simulink model "pneumatic_tank_PI"  (R2021a)
settings: Solver=VariableStepAuto  StartTime=0.0  StopTime=16  RelTol=1e-3
model workspace (MATLAB code in the model file):
  | V = 0.4; %liter
  | alpha = 1.5/3;
  | p_s = 6; % bar
values from neighbouring files (symbols this model uses):
  a = (Phi'*Phi)^(-1)*Phi'*p_dot    [sysid_tank.m]
  K = 2.62    [tank_valve_PI_design.m]
  p0 = 2.5    [tank_valve_PI_design.m]
undefined symbols (not defined in the file or in its folder): b, tau_i
settings Model: Creator=kjartan  LastModifiedBy=kjartan
settings SolverCC: AlgebraicLoopSolver=TrustRegion
settings DataIOCC: ReturnWorkspaceOutputs=off
settings DebuggingCC: SFMachineParentedDataDiag=warning  ArithmeticOperatorsInVariantConditions=warning
settings SFSimCC: CustomCodeUndefinedFunction=UseInterfaceOnly

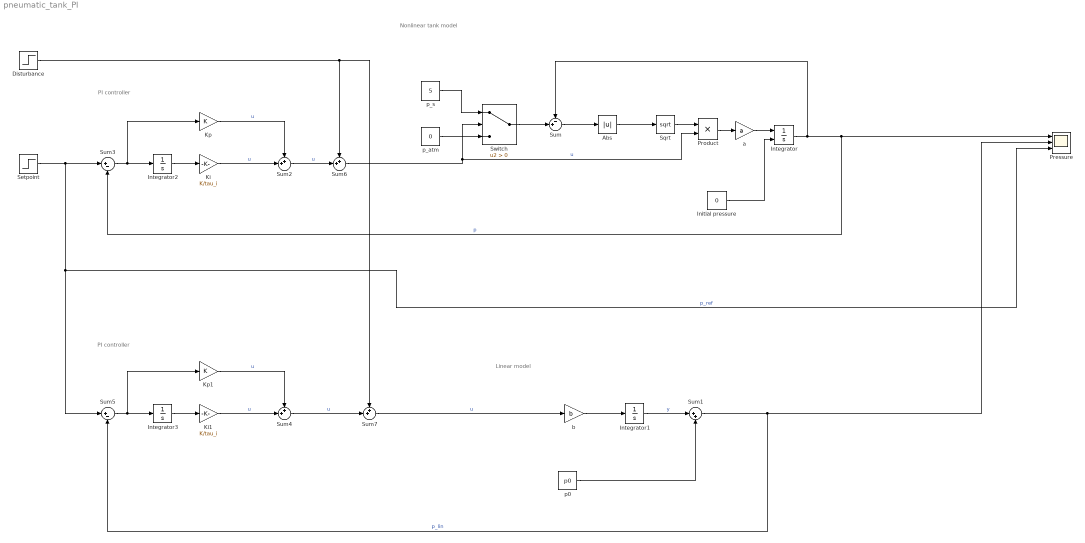
== system pneumatic_tank_PI ==
  note: PI controller
  note: PI controller
  note: Linear model
  note: Nonlinear tank model
  Abs : Abs
  Disturbance : Step  Time=10  SampleTime=0
  Initial pressure : Constant  Value=0  OutDataTypeStr=Inherit: Inherit via back propagation
  Integrator : Integrator  InitialConditionSource=external  InitialCondition=1  LimitOutput=on  LowerSaturationLimit=0
  Integrator1 : Integrator
  Integrator2 : Integrator
  Integrator3 : Integrator
  Ki : Gain  Gain=K/tau_i
  Ki1 : Gain  Gain=K/tau_i
  Kp : Gain  Gain=K
  Kp1 : Gain  Gain=K
  Pressure : Scope  NumInputPorts=3
  Product : Product
  Setpoint : Step  Time=2  After=4  SampleTime=0
  Sqrt : Sqrt  SaturateOnIntegerOverflow=on
  Sum : Sum  Inputs=-+|
  Sum1 : Sum  Inputs=|++
  Sum{2,4,6..7} (4 alike) : Sum  Inputs=++|
  Sum3 : Sum  Inputs=|+-
  Sum5 : Sum  Inputs=|+-
  Switch : Switch  Criteria=u2 > Threshold
  a : Gain  Gain=a
  b : Gain  Gain=b
  p0 : Constant  Value=p0
  p_atm : Constant  Value=0
  p_s : Constant  Value=5
  wires:
  Integrator/1 -> Sum/1, Sum3/2, Pressure/1  "p"
  Sum/1 -> Abs/1
  Sum6/1 -> Product/2, Switch/2  "u"
  a/1 -> Integrator/1
  Product/1 -> a/1
  p_s/1 -> Switch/1
  p_atm/1 -> Switch/3
  Switch/1 -> Sum/2
  Sqrt/1 -> Product/1
  Initial pressure/1 -> Integrator/2
  Abs/1 -> Sqrt/1
  b/1 -> Integrator1/1
  p0/1 -> Sum1/2
  Integrator1/1 -> Sum1/1  "y"
  Integrator2/1 -> Ki/1
  Ki/1 -> Sum2/2  "u"
  Kp/1 -> Sum2/1  "u"
  Sum3/1 -> Kp/1, Integrator2/1
  Sum1/1 -> Pressure/2, Sum5/2  "p_lin"
  Integrator3/1 -> Ki1/1
  Sum5/1 -> Kp1/1, Integrator3/1
  Sum7/1 -> b/1  "u"
  Kp1/1 -> Sum4/1  "u"
  Ki1/1 -> Sum4/2  "u"
  Setpoint/1 -> Pressure/3, Sum5/1, Sum3/1  "p_ref"
  Sum2/1 -> Sum6/2  "u"
  Disturbance/1 -> Sum7/1, Sum6/1
  Sum4/1 -> Sum7/2  "u"
